simulink model "QAM_16_dataAided_AGC_original"  (R2018a)
settings: Solver=ode45  StartTime=0.0  StopTime=1  RelTol=1e-3  EnableMultiTasking=on
values from neighbouring files (symbols this model uses):
  FrameTime = 0.000552    [qpsktxrx16.mat]
  qpsktxrx =     [qpsktxrx16.mat]
undefined symbols (not defined in the file or in its folder): dfilt
libraries: simulink x4, dspsigops x4, commdigbbndam3 x3, commblkintrlv2 x3, dspstat3 x3, dspobslib x3, commrflib2 x2, dspsrcs4 x2, commutil2 x2, commfilt2 x2, commchan3 x1, commblksprivate x1
(part 2 of 2)

== matlab function QAM_16_dataAided_AGC_original/Receiver/Fine Frequency Compensation/PED ==
  data: In input; e output
function e = PED(In)
% Implementation of Maximum Likelihood Phase Error Detector listed in
% Chapter 7.2.2 of "Digital Communications - A Discrete-Time Approach" by
% Michael Rice. This employs a decision directed method.
%
% Input:
%   In - Input samples, oversampled by two
% Output:
%   e - Phase error, de
%#codegen
M=16;
%for 64QAM constillation
if M==64

if real(In)>=0 && real(In)<2
    a=1;
elseif real(In)>=2 && real(In)<4
    a=3;
elseif real(In)>=4 && real(In)<6
    a=5;
elseif real(In)>=6
    a=7;
elseif real(In)<0 && real(In)>-2
    a=-1;
elseif real(In)<=-2 && real(In)>-4
    a=-3;
elseif real(In)<=-4 && real(In)>-6
    a=-5;
else
    a=-7;
end

if imag(In)>=0 && imag(In)<2
    b=1;
elseif imag(In)>=2 && imag(In)<4
    b=3;
elseif imag(In)>=4 && imag(In)<6
    b=5;
elseif imag(In)>=6
    b=7;
elseif imag(In)<0 && imag(In)>-2
    b=-1;
elseif imag(In)<=-2 && imag(In)>-4
    b=-3;
elseif imag(In)<=-4 && imag(In)>-6
    b=-5;
else
    b=-7;
end
r=sqrt(a^2+b^2);

%for 16QAM constillation
elseif M==16

if real(In)>=0 && real(In)<2
    a=1;
elseif real(In)>=2
    a=3;
elseif real(In)<0 && real(In)>=-2
    a=-1;
else
    a=-3;
end

if imag(In)>=0 && imag(In)<2
    b=1;
elseif imag(In)>=2
    b=3;
elseif imag(In)<0 && imag(In)>=-2
    b=-1;
else
    b=-3;

end
r=sqrt(a^2+b^2);

%for 4QAM constillation
else
r=1;

end

  
%R=sqrt(real(In)^2+imag(In)^2);
e =(sign(real(In)).*imag(In) - sign(imag(In)).*real(In))/r;






% function [error,I_hat,Q_hat] = PED(In)
% % Implementation of Maximum Likelihood Phase Error Detector listed in
% % Chapter 7.2.2 of "Digital Communications - A Discrete-Time Approach" by
% % Michael Rice. This employs a decision directed method.
% % 
% % Input: 
% %   In - Input samples, oversampled by two
% % Output:
% %   e - Phase error, de
% %#codegen
% 
% persistent e e1 e2 e3;
% if isempty(e1)
%     e = 0;
%     e1 = 0;
%     e2 = 0;
%     e3 = 0;
% end
% 
% if abs(real(In)) > 2
%     I_hat = sign(real(In))*3;
% else
%     I_hat = sign(real(In))*1;
% end
% 
% if abs(imag(In)) > 2
%     Q_hat = sign(imag(In))*3;
% else
%     Q_hat = sign(imag(In))*1;
% end
% 
% a = sqrt(I_hat^2 + Q_hat^2);
% b = sqrt(real(In)^2 + imag(In)^2);
% 
% if ((a~=0)&&(b~=0))
% e = ( ( I_hat.*imag(In) - Q_hat.*real(In) )/(a*b) );
% else 
%     e = 0;
% end;
% 
% %error = e;
% 
% if ((e> 0.8*e2) &&(e < 1.2*e2))
%     error = e;
% elseif ((e1> 0.8*e3) &&(e1 < 1.2*e3))
%     error = e1;
% else 
%     error = e;
% end
% 
% e3 = e2;
% e2 = e1;
% e1 = e;

== matlab function QAM_16_dataAided_AGC_original/Receiver/Timing Recovery/Timing Recovery PLL/Interpolation Filter ==
  data: In input; Out output; mu input
function Out = interp_filter(In, mu)
% Prabolic piecewise polynomial interpolator, Farrow Interpolator with 
% alpha = 1/2, see Figure 8.4.16 of "Digital Communications - A 
% Discrete-Time Approach" by Michael Rice.
% Input:
%   In - Input samples, oversampled by two
%   mu - Difference between actual sampling instant and the optimal instant,
%        between zero and one
% Output:
%   Out - Interpolation output
%#codegen
persistent delay1 delay2 delay3; % Input delayed by 1, 2 and 3 samples
if isempty(delay1)
    [delay1, delay2, delay3] = deal(complex(0,0));
end

K = -0.5;

Out = delay2 + mu.*(K.*(In+delay2+delay3)+(1-K).*delay1)...
      + K.*(delay1+delay2-In-delay3).*mu.^2;
  
% Update delay buffers
delay3 = delay2;
delay2 = delay1;
delay1 = In;

== matlab function QAM_16_dataAided_AGC_original/Receiver/Timing Recovery/Timing Recovery PLL/NCO Control ==
  data: Delta input; Underflow output; mu output; qpsktxrx parameter
function [Underflow, mu] = NCO_ctrl(Delta, qpsktxrx)
% Implementation of modulo-1 counter for interpolation control listed in
% Figure 8.4.19 of "Digital Communications - A Discrete-Time Approach"
% by Michael Rice. See design details in Chapter 8.4.3 of the same book.
% 
% Input:
%   Delta - Loop filter output. If loop is in lock, delta would be small
%   qpsktxrx - Simulation parameter structure
% Output:
%   Underflow - Indicator of counter underflow. This is the strobe signal
%   for downstream processing
%   mu - Difference between actual sampling instant and the optimal instant,
%        between zero and one
%#codegen

% delay1 - Counter value delayed by 1 sample
% Regtemp - The estimated timing error normalized by half QPSK symbols
persistent delay1 Regtemp;  
if isempty(delay1)
    [delay1, Regtemp] = deal(0);
end
Upsampling = qpsktxrx.Upsampling;
Downsampling = qpsktxrx.Downsampling;
oversampling = Upsampling/Downsampling;

counter = mod(delay1,1)-Delta-1/oversampling; % decrementing counter
if counter < 0
    Underflow = 1;
    Regtemp = mod(delay1,1)/(Delta+1/oversampling);
else
    Underflow = 0;
end

mu = Regtemp;

% Update delay buffer
delay1 = mod(delay1,1)-Delta-1/oversampling;

== matlab function QAM_16_dataAided_AGC_original/Receiver/Timing Recovery/Timing Recovery PLL/Timing Error Detector ==
  data: In input; e output; strobe input
function e = TED(In, strobe)
% Zero-Crossing Timing Error Detector. See "Zero-Crossing Timing Error
% Detector" section in Chapter 8.4.1 of "Digital Communications - A
% Discrete-Time Approach" by Michael Rice. For bit stuffing/stripping
% details, see page 490-494 of the same book.
%
% Input: 
%   In - Input samples, interpolation result
%   strobe - Signal to enable timing error calculation
% Output:
%   e - Timing error
%#codegen
persistent delay1 delay2 delayStrobe; % Input delayed by one and 2 samples, and
% Enable signal delayed by one sample
if isempty(delay1)
    [delay1, delay2] = deal(complex(0,0));
    delayStrobe = 0;
end

if strobe==1 && delayStrobe~=strobe
    e = real(delay1) * (sign(real(delay2)) - sign(real(In))) + ...
        imag(delay1) * (sign(imag(delay2)) - sign(imag(In)));
else
    e = 0;
end

if delayStrobe~=strobe
    % Shift contents in delay register
    delay2 = delay1;
    delay1 = In;
elseif strobe==1
    % Two consecutive high strobes
    delay2 = 0; % Stuff missing sample
    delay1 = In; 
end
% If both current and previous enable signals are 0, skip current sample
% and keep the delayed signals unchanged. (Bit stripping)
delayStrobe = strobe;

== matlab function QAM_16_dataAided_AGC_original/Receiver/Data Decoding/Align Data ==
  data: Delay input; RxData input; Data output
function Data  = aligndata(Delay, RxData)
% Extract data from the buffered RxData, using the delay to find the frame 


Data = RxData(Delay+1:Delay+length(RxData)/2);
